simulink model "ADHW4p3"  (R2022a)
settings: Solver=VariableStepAuto  StartTime=0.0  StopTime=1800.0  RelTol=1e-3
libraries: vrlib x1
settings Model: Creator=izacu  LastModifiedBy=izacu

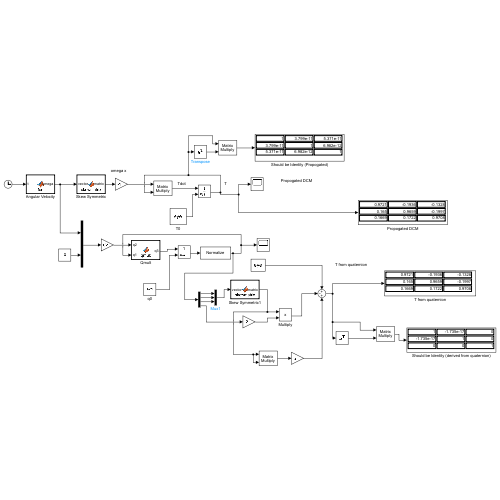
[thumbnail: Simulink's stored preview of the top-level diagram]
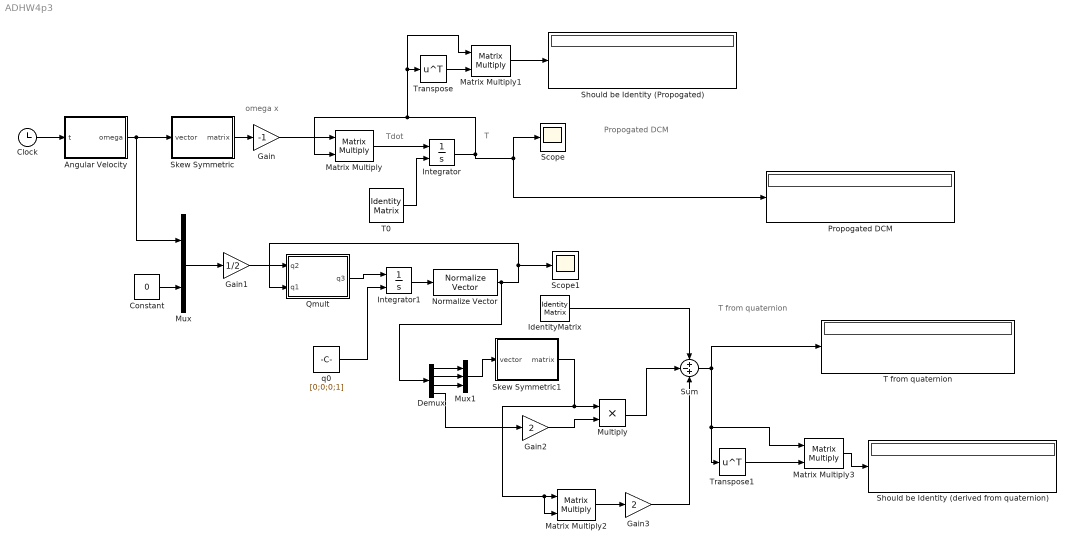
== system ADHW4p3 ==
  note: T from quaternion
  note: Propogated DCM
  note: Tdot
  note: T
  note: omega x
  Angular Velocity : MATLAB Function  TreatAsAtomicUnit=on
  Clock : Clock
  Constant : Constant  Value=0
  Demux : Demux
  Gain : Gain  Gain=-1
  Gain1 : Gain  Gain=1/2
  Gain2 : Gain  Gain=2
  Gain3 : Gain  Gain=2
  IdentityMatrix : IdentityMatrix  OutputDimensions=3
  Integrator : Integrator  InitialConditionSource=external
  Integrator1 : Integrator  InitialConditionSource=external
  Matrix Multiply{,1..3} (4 alike) : Product  Multiplication=Matrix(*)
  Multiply : Product  Inputs=**
  Mux : Mux  Inputs=2
  Mux1 : Mux  Inputs=3
  Normalize Vector : vrlib/Utilities/Normalize Vector  maxzero=0
  Propogated DCM : Display
  Qmult : MATLAB Function  TreatAsAtomicUnit=on
  Scope : Scope
  Scope1 : Scope
  Should be Identity (Propogated) : Display
  Should be Identity (derived from quaternion) : Display
  Skew Symmetric : MATLAB Function  TreatAsAtomicUnit=on
  Skew Symmetric1 : MATLAB Function  TreatAsAtomicUnit=on
  Sum : Sum  Inputs=+-+
  T from quaternion : Display
  T0 : IdentityMatrix  OutputDimensions=3
  Transpose : Math  Operator=transpose
  Transpose1 : Math  Operator=transpose
  q0 : Constant  Value=[0;0;0;1]
  wires:
  Clock/1 -> Angular Velocity/1(t)
  Angular Velocity/1(omega) -> Mux/1, Skew Symmetric/1(vector)
  T0/1 -> Integrator/2
  Skew Symmetric/1(matrix) -> Gain/1
  Gain/1 -> Matrix Multiply/1
  Integrator/1 -> Matrix Multiply1/1, Transpose/1, Matrix Multiply/2, Propogated DCM/1, Scope/1
  Matrix Multiply/1 -> Integrator/1
  Constant/1 -> Mux/2
  Mux/1 -> Gain1/1
  Gain1/1 -> Qmult/1(q2)
  Qmult/1(q3) -> Integrator1/1
  q0/1 -> Integrator1/2
  Integrator1/1 -> Normalize Vector/1
  Normalize Vector/1 -> Demux/1, Scope1/1, Qmult/2(q1)
  Transpose/1 -> Matrix Multiply1/2
  Matrix Multiply1/1 -> Should be Identity (Propogated)/1
  IdentityMatrix/1 -> Sum/1
  Demux/1 -> Mux1/1
  Demux/4 -> Gain2/1
  Skew Symmetric1/1(matrix) -> Matrix Multiply2/2, Matrix Multiply2/1, Multiply/1
  Gain2/1 -> Multiply/2
  Multiply/1 -> Sum/2
  Demux/2 -> Mux1/2
  Demux/3 -> Mux1/3
  Mux1/1 -> Skew Symmetric1/1(vector)
  Matrix Multiply2/1 -> Gain3/1
  Gain3/1 -> Sum/3
  Sum/1 -> Transpose1/1, Matrix Multiply3/1, T from quaternion/1
  Transpose1/1 -> Matrix Multiply3/2
  Matrix Multiply3/1 -> Should be Identity (derived from quaternion)/1

== matlab function ADHW4p3/Skew Symmetric ==
  data: vector input; matrix output
function matrix = skewmatrix(vector)

A = zeros(3,3);

A(1,2) = -vector(3);
A(1,3) = vector(2);
A(2,3) = -vector(1);
A(2,1) = vector(3);
A(3,1) = -vector(2);
A(3,2) = vector(1);

matrix = A;

== matlab function ADHW4p3/Angular Velocity ==
  data: t input; omega output
function omega = fcn(t)

omega = (2*pi/300)*[sin(2*pi*t/60); cos(2*pi*t/80); cos(2*pi*t/70)];

== matlab function ADHW4p3/Qmult ==
  data: q2 input; q1 input; q3 output
function q3 = qmult(q2,q1)

q3 = [q2(4).*q1(1:3) + q1(4).*q2(1:3) - cross(q2(1:3),q1(1:3));
    q2(4)*q1(4) - dot(q2(1:3),q1(1:3))];

== matlab function ADHW4p3/Skew Symmetric1 ==
  data: vector input; matrix output
function matrix = skewmatrix(vector)

A = zeros(3,3);

A(1,2) = -vector(3);
A(1,3) = vector(2);
A(2,3) = -vector(1);
A(2,1) = vector(3);
A(3,1) = -vector(2);
A(3,2) = vector(1);

matrix = A;
